simulink model "OFDM_Tx_Rx_InterpDec"  (R2020a)
settings: Solver=FixedStepDiscrete  StartTime=0.0  StopTime=inf  RelTol=1e-3
InitFcn:
  | % Set parameters
  | fs = 200e3;
  | 
  | % Load all required variables
  | load('read_addr_data');
  | load('read_addr_cp');
  | load('read_addr_pream');
  | load('read_addr_rx');
  | load('pilot');
  | load('LTSfreq');
  | load('STSfreq');
  | load('LTSread');
  | load('STSread');
  | load('bpsk');
  | load('qpsk');
  | load('qam16');
values from neighbouring files (symbols this model uses):
  bpsk = [0 0 1 1 1 1 0 0 1 0 1 0 ... (48 elements, 48x1)]    [bpsk.mat]
  qam16 = [12 5 10 3 14 8 1 10 8 7 2 13 ... (48 elements, 48x1)]    [qam16.mat]
  qpsk = [1 2 1 2 2 2 3 1 1 3 1 0 ... (48 elements, 48x1)]    [qpsk.mat]
  STSfreq = [0 0 0 0 0 0 0 0 1 0 0 0 ... (64 elements, 1x64)]    [STSfreq.mat]
undefined symbols (not defined in the file or in its folder): data3, designMultirateFIR, LTSfreq, LTSread, pilot, read_addr_cp, read_addr_data, read_addr_pream, read_addr_rx, STSread
libraries: hdlsllib x58, simulink x42, dspmlti4 x8, dsphdlxfrm x2, dsphdlmathfun x2, dsphdlsigops x1
(part 2 of 5)

== system OFDM_Tx_Rx_InterpDec/OFDMTx/ControlSignalGenerator/pilotValidGen ==
  enb : Inport
  AND : Logic  IconShape=distinctive  AllPortsSameDT=off  OutDataTypeStr=boolean
  Compare To Constant : simulink/Logic and Bit Operations/Compare To Constant  relop=<  const=32  OutDataTypeStr=boolean
  Compare To Constant1 : simulink/Logic and Bit Operations/Compare To Constant  relop=>  const=27  OutDataTypeStr=boolean
  HDL Counter : hdlsllib/Sources/HDL Counter  CountType=Count limited  CountInit=0  CountStep=1  CountMax=79  CountFromType=Initial value  CountFrom=0  CountResetPort=on  CountLoadPort=off  CountEnbPort=on  CountDirPort=off  CountDataType=Unsigned  CountWordLen=7  CountFracLen=0  CountSampTime=1
  NOT : Logic  Operator=NOT  IconShape=distinctive  AllPortsSameDT=off  OutDataTypeStr=boolean
  y : Outport
  wires:
  NOT/1 -> HDL Counter/1
  enb/1 -> HDL Counter/2, NOT/1
  HDL Counter/1 -> Compare To Constant1/1, Compare To Constant/1
  Compare To Constant/1 -> AND/1
  Compare To Constant1/1 -> AND/2
  AND/1 -> y/1

== system OFDM_Tx_Rx_InterpDec/OFDMTx/DataGenerator/LTSfreq ==
  preambVal : Inport
  AND : Logic  IconShape=distinctive  AllPortsSameDT=off  OutDataTypeStr=boolean
  AND1 : Logic  IconShape=distinctive  AllPortsSameDT=off  OutDataTypeStr=boolean
  Compare To Constant : simulink/Logic and Bit Operations/Compare To Constant  relop=>=  const=256  OutDataTypeStr=boolean
  Compare To Constant1 : simulink/Logic and Bit Operations/Compare To Constant  relop=<=  const=319  OutDataTypeStr=boolean
  HDL Counter1 : hdlsllib/Sources/HDL Counter  CountType=Count limited  CountInit=0  CountStep=1  CountMax=319  CountFromType=Initial value  CountFrom=0  CountResetPort=on  CountLoadPort=off  CountEnbPort=on  CountDirPort=off  CountDataType=Unsigned  CountWordLen=9  CountFracLen=0  CountSampTime=1
  HDL Counter4 : hdlsllib/Sources/HDL Counter  CountType=Count limited  CountInit=0  CountStep=1  CountMax=63  CountFromType=Initial value  CountFrom=0  CountResetPort=off  CountLoadPort=off  CountEnbPort=on  CountDirPort=off  CountDataType=Unsigned  CountWordLen=6  CountFracLen=0  CountSampTime=1
  LTSFreq : Lookup_n-D  NumberOfTableDimensions=1  LookupTableObject=''  BreakpointsForDimension1=0:63  BreakpointsForDimension1FirstPoint=10  BreakpointsForDimension2FirstPoint=10  BreakpointsForDimension1Spacing=12  BreakpointsForDimension2Spacing=12  IndexSearchMethod=Evenly spaced points  Table=LTSfreq  TableDataTypeStr=fixdt(1,16,14)  InterpMethod=Flat  DiagnosticForOutOfRangeInput=Error  InternalRulePriority=Speed  OutDataTypeStr=fixdt(1,16,14)  RndMeth=Simplest  InputSameDT=on
  NOT : Logic  Operator=NOT  IconShape=distinctive  AllPortsSameDT=off  OutDataTypeStr=boolean
  ltsFreq : Outport  VectorParamsAs1DForOutWhenUnconnected=off
  ltsVal : Outport  Port=2  VectorParamsAs1DForOutWhenUnconnected=off
  wires:
  HDL Counter4/1 -> LTSFreq/1
  Compare To Constant/1 -> AND/1
  HDL Counter1/1 -> Compare To Constant1/1, Compare To Constant/1
  Compare To Constant1/1 -> AND/2
  NOT/1 -> HDL Counter1/1
  AND/1 -> AND1/1
  preambVal/1 -> NOT/1, AND1/2, HDL Counter1/2
  AND1/1 -> ltsVal/1, HDL Counter4/1
  LTSFreq/1 -> ltsFreq/1

== system OFDM_Tx_Rx_InterpDec/OFDMTx/DataGenerator/PilotGen ==
  dataValidIn : Inport
  pilotValidIn : Inport  Port=2
  Compare To Constant : simulink/Logic and Bit Operations/Compare To Constant  relop=>  const=0  OutDataTypeStr=boolean
  Compare To Constant1 : simulink/Logic and Bit Operations/Compare To Constant  relop===  const=79  OutDataTypeStr=boolean
  Constant : Constant  Value=0  OutDataTypeStr=fixdt(1,2,0)  SampleTime=1/fs
  Data Type Conversion1 : DataTypeConversion  OutDataTypeStr=fixdt(1,16,14)
  HDL Counter : hdlsllib/Sources/HDL Counter  CountType=Count limited  CountInit=0  CountStep=1  CountMax=3  CountFromType=Initial value  CountFrom=0  CountResetPort=off  CountLoadPort=off  CountEnbPort=on  CountDirPort=off  CountDataType=Unsigned  CountWordLen=2  CountFracLen=0  CountSampTime=1
  HDL Counter1 : hdlsllib/Sources/HDL Counter  CountType=Count limited  CountInit=0  CountStep=1  CountMax=79  CountFromType=Initial value  CountFrom=0  CountResetPort=on  CountLoadPort=off  CountEnbPort=on  CountDirPort=off  CountDataType=Unsigned  CountWordLen=8  CountFracLen=0  CountSampTime=1
  HDL Counter2 : hdlsllib/Sources/HDL Counter  CountType=Count limited  CountInit=0  CountStep=1  CountMax=126  CountFromType=Initial value  CountFrom=0  CountResetPort=on  CountLoadPort=off  CountEnbPort=on  CountDirPort=off  CountDataType=Unsigned  CountWordLen=7  CountFracLen=0  CountSampTime=1
  NOT : Logic  Operator=NOT  IconShape=distinctive  AllPortsSameDT=off  OutDataTypeStr=boolean
  PilotValue_LUT : Lookup_n-D  NumberOfTableDimensions=1  LookupTableObject=''  BreakpointsForDimension1=[0:3]  BreakpointsForDimension1FirstPoint=10  BreakpointsForDimension2FirstPoint=10  BreakpointsForDimension1Spacing=12  BreakpointsForDimension2Spacing=12  IndexSearchMethod=Evenly spaced points  Table=[1 1 1 -1]  TableDataTypeStr=fixdt(1,2,0)  InterpMethod=Flat  DiagnosticForOutOfRangeInput=Error  InternalRulePriority=Speed  OutDataTypeStr=fixdt(1,2,0)  RndMeth=Simplest  InputSameDT=on
  Polarity_LUT : Lookup_n-D  NumberOfTableDimensions=1  LookupTableObject=''  BreakpointsForDimension1=[0:126]  BreakpointsForDimension1FirstPoint=10  BreakpointsForDimension2FirstPoint=10  BreakpointsForDimension1Spacing=12  BreakpointsForDimension2Spacing=12  IndexSearchMethod=Evenly spaced points  Table=pilot  TableDataTypeStr=fixdt(1,2,0)  InterpMethod=Flat  DiagnosticForOutOfRangeInput=Error  InternalRulePriority=Speed  OutDataTypeStr=fixdt(1,2,0)  RndMeth=Simplest  InputSameDT=on
  Switch : Switch  Criteria=u2 ~= 0
  Switch1 : Switch  Criteria=u2 ~= 0
  ToComplex1 : Subsystem
  Unary Minus : UnaryMinus
  pilotOut : Outport  VectorParamsAs1DForOutWhenUnconnected=off
  wires:
  HDL Counter/1 -> PilotValue_LUT/1
  Data Type Conversion1/1 -> ToComplex1/1(In1)
  dataValidIn/1 -> HDL Counter1/2, NOT/1
  HDL Counter1/1 -> Compare To Constant1/1
  NOT/1 -> HDL Counter2/1, HDL Counter1/1
  Compare To Constant1/1 -> HDL Counter2/2
  HDL Counter2/1 -> Polarity_LUT/1
  ToComplex1/1(PilotOut) -> pilotOut/1
  pilotValidIn/1 -> HDL Counter/1, Switch1/2
  Polarity_LUT/1 -> Compare To Constant/1
  Compare To Constant/1 -> Switch/2
  Unary Minus/1 -> Switch/3
  Switch/1 -> Data Type Conversion1/1
  PilotValue_LUT/1 -> Switch1/1
  Switch1/1 -> Unary Minus/1, Switch/1
  Constant/1 -> Switch1/3

== system OFDM_Tx_Rx_InterpDec/OFDMTx/DataGenerator/STSFreq ==
  preamVal : Inport
  AND : Logic  IconShape=distinctive  AllPortsSameDT=off  OutDataTypeStr=boolean
  AND1 : Logic  IconShape=distinctive  AllPortsSameDT=off  OutDataTypeStr=boolean
  Compare To Constant : simulink/Logic and Bit Operations/Compare To Constant  relop=>=  const=96  OutDataTypeStr=boolean
  Compare To Constant1 : simulink/Logic and Bit Operations/Compare To Constant  relop=<=  const=159  OutDataTypeStr=boolean
  HDL Counter : hdlsllib/Sources/HDL Counter  CountType=Count limited  CountInit=0  CountStep=1  CountMax=63  CountFromType=Initial value  CountFrom=0  CountResetPort=off  CountLoadPort=off  CountEnbPort=on  CountDirPort=off  CountDataType=Unsigned  CountWordLen=6  CountFracLen=0  CountSampTime=1
  HDL Counter1 : hdlsllib/Sources/HDL Counter  CountType=Count limited  CountInit=0  CountStep=1  CountMax=319  CountFromType=Initial value  CountFrom=0  CountResetPort=on  CountLoadPort=off  CountEnbPort=on  CountDirPort=off  CountDataType=Unsigned  CountWordLen=9  CountFracLen=0  CountSampTime=1
  NOT : Logic  Operator=NOT  IconShape=distinctive  AllPortsSameDT=off  OutDataTypeStr=boolean
  STSFreq : Lookup_n-D  NumberOfTableDimensions=1  LookupTableObject=''  BreakpointsForDimension1=[0:63]  BreakpointsForDimension1FirstPoint=10  BreakpointsForDimension2FirstPoint=10  BreakpointsForDimension1Spacing=12  BreakpointsForDimension2Spacing=12  IndexSearchMethod=Evenly spaced points  Table=STSfreq  TableDataTypeStr=fixdt(1,16,14)  InterpMethod=Flat  DiagnosticForOutOfRangeInput=Error  InternalRulePriority=Speed  OutDataTypeStr=fixdt(1,16,14)  RndMeth=Simplest  InputSameDT=on
  stsFreq : Outport  VectorParamsAs1DForOutWhenUnconnected=off
  stsVal : Outport  Port=2  VectorParamsAs1DForOutWhenUnconnected=off
  wires:
  HDL Counter/1 -> STSFreq/1
  AND/1 -> AND1/1
  HDL Counter1/1 -> Compare To Constant1/1, Compare To Constant/1
  NOT/1 -> HDL Counter1/1
  Compare To Constant/1 -> AND/1
  Compare To Constant1/1 -> AND/2
  preamVal/1 -> NOT/1, AND1/2, HDL Counter1/2
  AND1/1 -> stsVal/1, HDL Counter/1
  STSFreq/1 -> stsFreq/1

== system OFDM_Tx_Rx_InterpDec/OFDMTx/DataGenerator/SymbolsGen ==
  modScheme : Inport
  valid : Inport  Port=2
  BPSKmap : Subsystem
  DataGenerator : Subsystem
  DataGenerator1 : Subsystem
  DataGenerator2 : Subsystem  Commented=on
  DataGenerator3 : Subsystem
  Multiport Switch : MultiPortSwitch  DataPortOrder=Zero-based contiguous  zeroidx=on
  QPSKMap : Subsystem
  QPSKMap1 : Subsystem
  symbsOut : Outport  VectorParamsAs1DForOutWhenUnconnected=off
  wires:
  BPSKmap/1(BPSKOut) -> Multiport Switch/2
  modScheme/1 -> Multiport Switch/1
  Multiport Switch/1 -> symbsOut/1
  QPSKMap/1(QPSKOut) -> Multiport Switch/3
  QPSKMap1/1(16QAM) -> Multiport Switch/4
  DataGenerator3/1(bits) -> QPSKMap1/1(ints)
  DataGenerator3/2(validOut) -> QPSKMap1/2(validIn)
  DataGenerator1/1(bits) -> QPSKMap/1(ints)
  DataGenerator1/2(validOut) -> QPSKMap/2(validIn)
  DataGenerator/1(bits) -> BPSKmap/1(bits)
  DataGenerator/2(validOut) -> BPSKmap/2(validIn)
  valid/1 -> DataGenerator3/1(ready), DataGenerator1/1(ready), DataGenerator/1(ready)

== system OFDM_Tx_Rx_InterpDec/OFDMTx/IFFT/IFFTValid ==
  preambleValid : Inport
  dataValid : Inport  Port=2
  Switch : Switch  Criteria=u2 ~= 0
  dataIFFTValid : Subsystem
  preambIFFTValid : Subsystem
  ifftValid : Outport  VectorParamsAs1DForOutWhenUnconnected=off
  wires:
  preambleValid/1 -> Switch/2, preambIFFTValid/1(preambValid)
  preambIFFTValid/1(preambIFFTValidOut) -> Switch/1
  dataValid/1 -> dataIFFTValid/1(dataValidIn)
  dataIFFTValid/1(dataIFFTValidOut) -> Switch/3
  Switch/1 -> ifftValid/1

== system OFDM_Tx_Rx_InterpDec/OFDMTx/SCMapper/DataMapper ==
  dataIn : Inport
  dataValid : Inport  Port=2
  Delay1 : Delay  DelayLength=80  InitialCondition=0  UseCircularBuffer=on
  Delay2 : Delay  DelayLength=80
  Delay3 : Delay  DelayLength=1  InitialCondition=0  UseCircularBuffer=on
  Delay4 : Delay  DelayLength=80
  Dual Port RAM2 : hdlsllib/HDL RAMs/Dual Port RAM  ram_size=8
      settings: SourceProductBaseCode=SL
  HDL Counter : hdlsllib/Sources/HDL Counter  CountType=Count limited  CountInit=0  CountStep=1  CountMax=159  CountFromType=Initial value  CountFrom=0  CountResetPort=off  CountLoadPort=off  CountEnbPort=on  CountDirPort=off  CountDataType=Unsigned  CountWordLen=8  CountFracLen=0  CountSampTime=1
  HDL Counter1 : hdlsllib/Sources/HDL Counter  CountType=Count limited  CountInit=0  CountStep=1  CountMax=159  CountFromType=Initial value  CountFrom=0  CountResetPort=off  CountLoadPort=off  CountEnbPort=on  CountDirPort=off  CountDataType=Unsigned  CountWordLen=8  CountFracLen=0  CountSampTime=1
  READ_CTRL2 : Subsystem
  Terminator3 : Terminator
  readaddress : Lookup_n-D  NumberOfTableDimensions=1  LookupTableObject=''  BreakpointsForDimension1=[0:159]  BreakpointsForDimension1FirstPoint=10  BreakpointsForDimension2FirstPoint=10  BreakpointsForDimension1Spacing=12  BreakpointsForDimension2Spacing=12  IndexSearchMethod=Evenly spaced points  Table=read_addr_data  TableDataTypeStr=fixdt(0,8,0)  InterpMethod=Flat  DiagnosticForOutOfRangeInput=Error  InternalRulePriority=Speed  OutDataTypeStr=fixdt(0,8,0)  RndMeth=Simplest  InputSameDT=on
  dataOut : Outport  VectorParamsAs1DForOutWhenUnconnected=off
  dataValidOut : Outport  Port=2  VectorParamsAs1DForOutWhenUnconnected=off
  wires:
  READ_CTRL2/1(Out1) -> Dual Port RAM2/4
  Delay3/1 -> Delay2/1
  dataValid/1 -> HDL Counter1/1, Delay1/1, Dual Port RAM2/3
  Dual Port RAM2/2 -> Delay4/1
  Delay1/1 -> READ_CTRL2/2(In2), Delay3/1, HDL Counter/1
  HDL Counter1/1 -> Dual Port RAM2/2
  dataIn/1 -> Dual Port RAM2/1
  HDL Counter/1 -> readaddress/1
  readaddress/1 -> READ_CTRL2/1(In1)
  Dual Port RAM2/1 -> Terminator3/1
  Delay2/1 -> dataValidOut/1
  Delay4/1 -> dataOut/1

== system OFDM_Tx_Rx_InterpDec/OFDMTx/SCMapper/PremableMapper ==
  data : Inport
  preambVal : Inport  Port=2
  Delay : Delay  DelayLength=160  InitialCondition=0  UseCircularBuffer=on
  Delay12 : Delay  DelayLength=1  InitialCondition=0  UseCircularBuffer=on
  Dual Port RAM : hdlsllib/HDL RAMs/Dual Port RAM  ram_size=9
      settings: SourceProductBaseCode=SL
  HDL Counter2 : hdlsllib/Sources/HDL Counter  CountType=Count limited  CountInit=0  CountStep=1  CountMax=319  CountFromType=Initial value  CountFrom=0  CountResetPort=off  CountLoadPort=off  CountEnbPort=on  CountDirPort=off  CountDataType=Unsigned  CountWordLen=9  CountFracLen=0  CountSampTime=1
  HDL Counter3 : hdlsllib/Sources/HDL Counter  CountType=Count limited  CountInit=0  CountStep=1  CountMax=319  CountFromType=Initial value  CountFrom=0  CountResetPort=off  CountLoadPort=off  CountEnbPort=on  CountDirPort=off  CountDataType=Unsigned  CountWordLen=9  CountFracLen=0  CountSampTime=1
  READ_CTRL : Subsystem
  Terminator1 : Terminator
  readaddr : Lookup_n-D  NumberOfTableDimensions=1  LookupTableObject=''  BreakpointsForDimension1=0:319  BreakpointsForDimension1FirstPoint=10  BreakpointsForDimension2FirstPoint=10  BreakpointsForDimension1Spacing=12  BreakpointsForDimension2Spacing=12  IndexSearchMethod=Evenly spaced points  Table=read_addr_pream  TableDataTypeStr=fixdt(0,9,0)  InterpMethod=Flat  DiagnosticForOutOfRangeInput=Error  InternalRulePriority=Speed  OutDataTypeStr=fixdt(0,9,0)  RndMeth=Simplest  InputSameDT=on
  preambleShiftOut : Outport  VectorParamsAs1DForOutWhenUnconnected=off
  preambValOut : Outport  Port=2  VectorParamsAs1DForOutWhenUnconnected=off
  wires:
  readaddr/1 -> READ_CTRL/1(In1)
  preambVal/1 -> Delay/1, Dual Port RAM/3, HDL Counter3/1
  READ_CTRL/1(Out1) -> Dual Port RAM/4
  HDL Counter3/1 -> Dual Port RAM/2
  Delay/1 -> READ_CTRL/2(In2), Delay12/1, HDL Counter2/1
  Dual Port RAM/1 -> Terminator1/1
  Delay12/1 -> preambValOut/1
  HDL Counter2/1 -> readaddr/1
  data/1 -> Dual Port RAM/1
  Dual Port RAM/2 -> preambleShiftOut/1

== system OFDM_Tx_Rx_InterpDec/OFDMRx/ChannelEstEq/ChannelEstimate/ChanEst ==
  note: Store conjugate as this is used in the
      | equaliser.
  note: Read out frequency domain LTS
      | when preamble valid is HIGH and
      | use this to obtain channel estimate.
  note: 1st half
  note: 2nd half
  ChanEstIn : Inport
  PreambValidIn : Inport  Port=2
  Delay : Delay  DelayLength=64
  Delay{1..7} (7 alike) : Delay  DelayLength=1
  Gain : Gain  Gain=0.5  OutDataTypeStr=fixdt(1,17,14)
  HDL Counter : hdlsllib/Sources/HDL Counter  CountType=Count limited  CountInit=0  CountStep=1  CountMax=63  CountFromType=Initial value  CountFrom=0  CountResetPort=off  CountLoadPort=off  CountEnbPort=on  CountDirPort=off  CountDataType=Unsigned  CountWordLen=6  CountFracLen=0  CountSampTime=1
  InvLLTF : Lookup_n-D  NumberOfTableDimensions=1  BreakpointsForDimension1=0:63  IndexSearchMethod=Evenly spaced points  Table=fftshift(LTSfreq)  TableDataTypeStr=fixdt(1,16,0)  InterpMethod=Flat  ExtrapMethod=Clip  UseLastTableValue=on  InternalRulePriority=Speed  OutDataTypeStr=fixdt(1,16,0)  RndMeth=Simplest  InputSameDT=on
  Math Function : Math  Operator=conj  SignedPower=on  SaturateOnIntegerOverflow=on
  Product : Product  OutDataTypeStr=fixdt(1,16,14)
  Subtract : Sum
  ChEstOut : Outport  VectorParamsAs1DForOutWhenUnconnected=off
  wires:
  Delay7/1 -> Math Function/1
  Delay6/1 -> Subtract/2, Delay/1
  Delay5/1 -> Product/2
  InvLLTF/1 -> Delay5/1
  Delay4/1 -> Product/1
  HDL Counter/1 -> InvLLTF/1
  Gain/1 -> Delay7/1
  Product/1 -> Delay6/1
  Delay/1 -> Subtract/1
  Math Function/1 -> Delay3/1
  ChanEstIn/1 -> Delay1/1
  PreambValidIn/1 -> Delay2/1
  Delay1/1 -> Delay4/1
  Delay2/1 -> HDL Counter/1
  Delay3/1 -> ChEstOut/1
  Subtract/1 -> Gain/1

== system OFDM_Tx_Rx_InterpDec/OFDMRx/ChannelEstEq/ChannelEstimate/WriteEnbAddrGen ==
  In1 : Inport
  AND : Logic  IconShape=distinctive  AllPortsSameDT=off  OutDataTypeStr=boolean
  Compare To Constant : simulink/Logic and Bit Operations/Compare To Constant  relop=>=  const=64  OutDataTypeStr=boolean
  Compare To Constant1 : simulink/Logic and Bit Operations/Compare To Constant  relop=<=  const=127  OutDataTypeStr=boolean
  HDL Counter1 : hdlsllib/Sources/HDL Counter  CountType=Count limited  CountInit=0  CountStep=1  CountMax=63  CountFromType=Initial value  CountFrom=0  CountResetPort=off  CountLoadPort=off  CountEnbPort=on  CountDirPort=off  CountDataType=Unsigned  CountWordLen=6  CountFracLen=0  CountSampTime=1
  HDL Counter2 : hdlsllib/Sources/HDL Counter  CountType=Count limited  CountInit=0  CountStep=1  CountMax=127  CountFromType=Initial value  CountFrom=0  CountResetPort=off  CountLoadPort=off  CountEnbPort=on  CountDirPort=off  CountDataType=Unsigned  CountWordLen=7  CountFracLen=0  CountSampTime=1
  Out1 : Outport  VectorParamsAs1DForOutWhenUnconnected=off
  Out2 : Outport  Port=2  VectorParamsAs1DForOutWhenUnconnected=off
  wires:
  In1/1 -> HDL Counter2/1
  HDL Counter2/1 -> Compare To Constant/1, Compare To Constant1/1
  AND/1 -> Out2/1, HDL Counter1/1
  HDL Counter1/1 -> Out1/1
  Compare To Constant/1 -> AND/1
  Compare To Constant1/1 -> AND/2

== system OFDM_Tx_Rx_InterpDec/OFDMRx/ChannelEstEq/Equalise/Abs2 ==
  ChEstIn : Inport
  Add : Sum  OutDataTypeStr=fixdt(0,16,14)
  Complex to Real-Imag : ComplexToRealImag
  Delay{,1..4} (5 alike) : Delay  DelayLength=1
  Product : Product
  Product1 : Product
  Out1 : Outport  VectorParamsAs1DForOutWhenUnconnected=off
  wires:
  Delay3/1 -> Add/2
  Delay2/1 -> Add/1
  Delay1/1 -> Product1/1, Product1/2
  Delay/1 -> Product/2, Product/1
  Complex to Real-Imag/2 -> Delay1/1
  Product1/1 -> Delay3/1
  Product/1 -> Delay2/1
  ChEstIn/1 -> Complex to Real-Imag/1
  Complex to Real-Imag/1 -> Delay/1
  Add/1 -> Delay4/1
  Delay4/1 -> Out1/1

== system OFDM_Tx_Rx_InterpDec/OFDMRx/ChannelEstEq/Equalise/Complex Mult ==
  In1 : Inport
  In2 : Inport  Port=2
  Delay4 : Delay  DelayLength=1
  Delay5 : Delay  DelayLength=1
  Delay7 : Delay
  Product1 : Product  OutDataTypeStr=fixdt(1,18,15)
  Out1 : Outport
  wires:
  Product1/1 -> Delay7/1
  Delay4/1 -> Product1/1
  In1/1 -> Delay4/1
  Delay5/1 -> Product1/2
  Delay7/1 -> Out1/1
  In2/1 -> Delay5/1

== system OFDM_Tx_Rx_InterpDec/OFDMRx/ChannelEstEq/Equalise/Divide ==
  In1 : Inport
  In2 : Inport  Port=2
  Delay1 : Delay  DelayLength=1
  Delay2 : Delay  DelayLength=1
  Delay8 : Delay  DelayLength=1
  Product2 : Product  OutDataTypeStr=fixdt(1,18,15)
  Reciprocal : Product  Inputs=/  OutDataTypeStr=fixdt(0,25,15)  RndMeth=Zero  SaturateOnIntegerOverflow=on
  Out1 : Outport
  wires:
  Reciprocal/1 -> Delay1/1
  In2/1 -> Reciprocal/1
  In1/1 -> Delay8/1
  Delay8/1 -> Product2/1
  Delay1/1 -> Product2/2
  Product2/1 -> Delay2/1
  Delay2/1 -> Out1/1

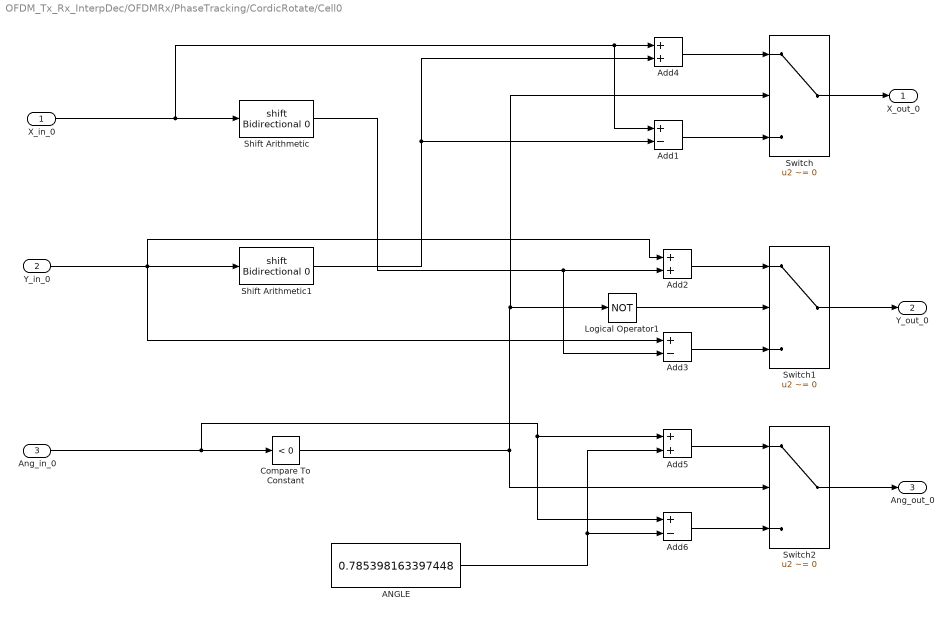
== system OFDM_Tx_Rx_InterpDec/OFDMRx/PhaseTracking/CordicRotate/Cell0 ==
  X_in_0 : Inport
  Y_in_0 : Inport  Port=2
  Ang_in_0 : Inport  Port=3
  ANGLE : Constant  Value=0.785398163397448  VectorParams1D=off  OutDataTypeStr=fixdt(1,23,20)  SampleTime=1/fs
  Add1 : Sum  Inputs=+-  OutDataTypeStr=fixdt(1,21,15)
  Add2 : Sum  OutDataTypeStr=fixdt(1,21,15)
  Add3 : Sum  Inputs=+-  OutDataTypeStr=fixdt(1,21,15)
  Add4 : Sum  OutDataTypeStr=fixdt(1,21,15)
  Add5 : Sum  OutDataTypeStr=fixdt(1,23,20)
  Add6 : Sum  Inputs=+-  OutDataTypeStr=fixdt(1,23,20)
  Compare To Constant : simulink/Logic and Bit Operations/Compare To Constant  relop=<  const=0  OutDataTypeStr=boolean
  Logical Operator1 : Logic  Operator=NOT  IconShape=distinctive  AllPortsSameDT=off  OutDataTypeStr=boolean
  Shift Arithmetic : ArithShift
  Shift Arithmetic1 : ArithShift
  Switch : Switch  Criteria=u2 ~= 0
  Switch1 : Switch  Criteria=u2 ~= 0
  Switch2 : Switch  Criteria=u2 ~= 0
  X_out_0 : Outport  VectorParamsAs1DForOutWhenUnconnected=off
  Y_out_0 : Outport  Port=2  VectorParamsAs1DForOutWhenUnconnected=off
  Ang_out_0 : Outport  Port=3  VectorParamsAs1DForOutWhenUnconnected=off
  wires:
  ANGLE/1 -> Add5/2, Add6/2
  Logical Operator1/1 -> Switch1/2
  Shift Arithmetic/1 -> Add2/2, Add3/2
  Shift Arithmetic1/1 -> Add4/2, Add1/2
  Compare To Constant/1 -> Switch2/2, Switch/2, Logical Operator1/1
  Ang_in_0/1 -> Compare To Constant/1, Add5/1, Add6/1
  Y_in_0/1 -> Add2/1, Add3/1, Shift Arithmetic1/1
  X_in_0/1 -> Add4/1, Add1/1, Shift Arithmetic/1
  Switch2/1 -> Ang_out_0/1
  Add5/1 -> Switch2/1
  Add6/1 -> Switch2/3
  Switch1/1 -> Y_out_0/1
  Switch/1 -> X_out_0/1
  Add2/1 -> Switch1/1
  Add3/1 -> Switch1/3
  Add1/1 -> Switch/3
  Add4/1 -> Switch/1

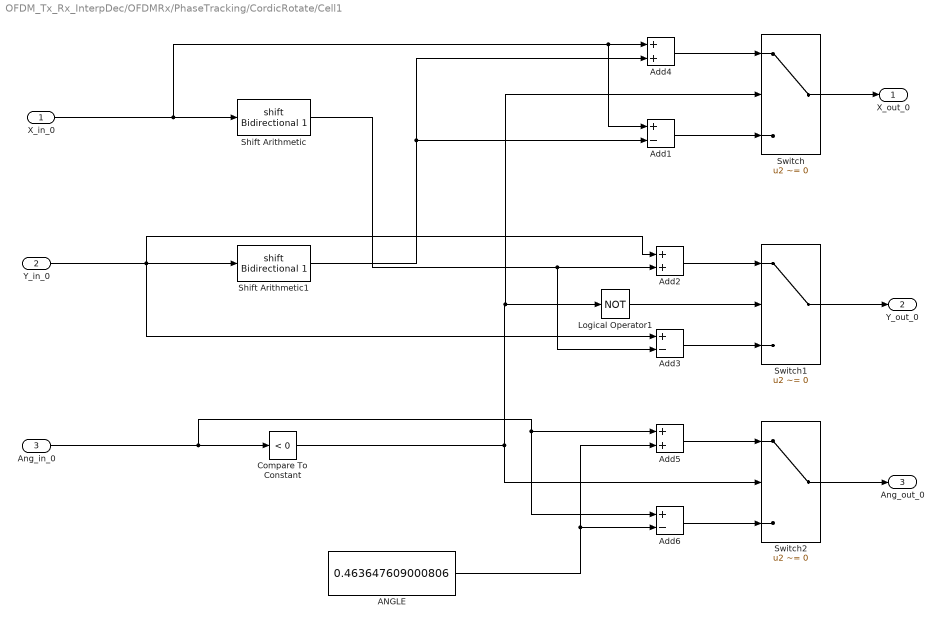
== system OFDM_Tx_Rx_InterpDec/OFDMRx/PhaseTracking/CordicRotate/Cell1 ==
  X_in_0 : Inport
  Y_in_0 : Inport  Port=2
  Ang_in_0 : Inport  Port=3
  ANGLE : Constant  Value=0.463647609000806  VectorParams1D=off  OutDataTypeStr=fixdt(1,23,20)  SampleTime=1/fs
  Add1 : Sum  Inputs=+-  OutDataTypeStr=fixdt(1,21,15)
  Add2 : Sum  OutDataTypeStr=fixdt(1,21,15)
  Add3 : Sum  Inputs=+-  OutDataTypeStr=fixdt(1,21,15)
  Add4 : Sum  OutDataTypeStr=fixdt(1,21,15)
  Add5 : Sum  OutDataTypeStr=fixdt(1,23,20)
  Add6 : Sum  Inputs=+-  OutDataTypeStr=fixdt(1,23,20)
  Compare To Constant : simulink/Logic and Bit Operations/Compare To Constant  relop=<  const=0  OutDataTypeStr=boolean
  Logical Operator1 : Logic  Operator=NOT  IconShape=distinctive  AllPortsSameDT=off  OutDataTypeStr=boolean
  Shift Arithmetic : ArithShift  BitShiftNumber=1
  Shift Arithmetic1 : ArithShift  BitShiftNumber=1
  Switch : Switch  Criteria=u2 ~= 0
  Switch1 : Switch  Criteria=u2 ~= 0
  Switch2 : Switch  Criteria=u2 ~= 0
  X_out_0 : Outport  VectorParamsAs1DForOutWhenUnconnected=off
  Y_out_0 : Outport  Port=2  VectorParamsAs1DForOutWhenUnconnected=off
  Ang_out_0 : Outport  Port=3  VectorParamsAs1DForOutWhenUnconnected=off
  wires:
  Add4/1 -> Switch/1
  Add1/1 -> Switch/3
  Add3/1 -> Switch1/3
  Add2/1 -> Switch1/1
  Switch/1 -> X_out_0/1
  Switch1/1 -> Y_out_0/1
  Add6/1 -> Switch2/3
  Add5/1 -> Switch2/1
  Switch2/1 -> Ang_out_0/1
  X_in_0/1 -> Shift Arithmetic/1, Add1/1, Add4/1
  Y_in_0/1 -> Shift Arithmetic1/1, Add3/1, Add2/1
  Ang_in_0/1 -> Add6/1, Add5/1, Compare To Constant/1
  Compare To Constant/1 -> Logical Operator1/1, Switch/2, Switch2/2
  Shift Arithmetic1/1 -> Add1/2, Add4/2
  Shift Arithmetic/1 -> Add3/2, Add2/2
  Logical Operator1/1 -> Switch1/2
  ANGLE/1 -> Add6/2, Add5/2

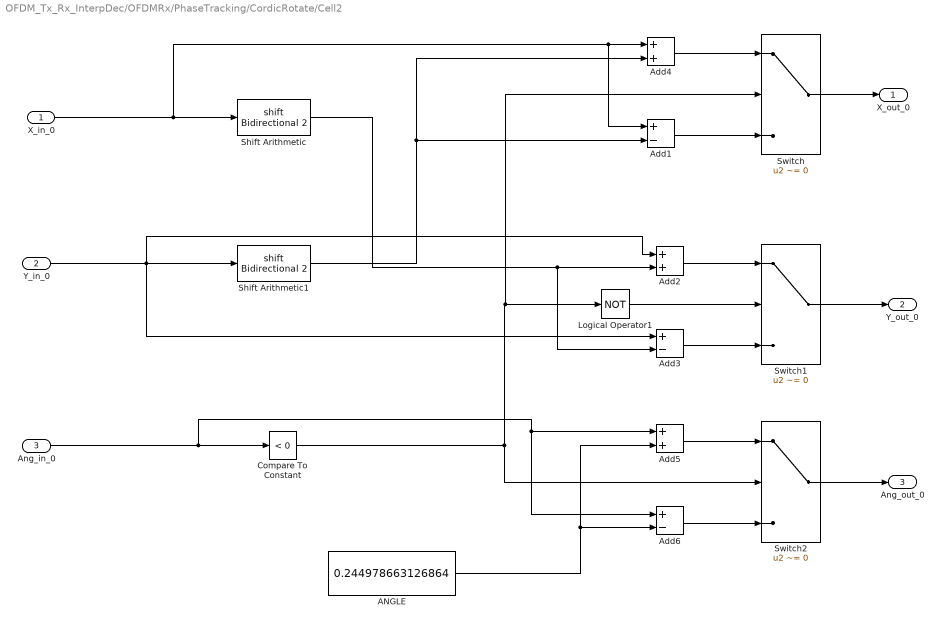
== system OFDM_Tx_Rx_InterpDec/OFDMRx/PhaseTracking/CordicRotate/Cell2 ==
  X_in_0 : Inport
  Y_in_0 : Inport  Port=2
  Ang_in_0 : Inport  Port=3
  ANGLE : Constant  Value=0.244978663126864  VectorParams1D=off  OutDataTypeStr=fixdt(1,23,20)  SampleTime=1/fs
  Add1 : Sum  Inputs=+-  OutDataTypeStr=fixdt(1,21,15)
  Add2 : Sum  OutDataTypeStr=fixdt(1,21,15)
  Add3 : Sum  Inputs=+-  OutDataTypeStr=fixdt(1,21,15)
  Add4 : Sum  OutDataTypeStr=fixdt(1,21,15)
  Add5 : Sum  OutDataTypeStr=fixdt(1,23,20)
  Add6 : Sum  Inputs=+-  OutDataTypeStr=fixdt(1,23,20)
  Compare To Constant : simulink/Logic and Bit Operations/Compare To Constant  relop=<  const=0  OutDataTypeStr=boolean
  Logical Operator1 : Logic  Operator=NOT  IconShape=distinctive  AllPortsSameDT=off  OutDataTypeStr=boolean
  Shift Arithmetic : ArithShift  BitShiftNumber=2
  Shift Arithmetic1 : ArithShift  BitShiftNumber=2
  Switch : Switch  Criteria=u2 ~= 0
  Switch1 : Switch  Criteria=u2 ~= 0
  Switch2 : Switch  Criteria=u2 ~= 0
  X_out_0 : Outport  VectorParamsAs1DForOutWhenUnconnected=off
  Y_out_0 : Outport  Port=2  VectorParamsAs1DForOutWhenUnconnected=off
  Ang_out_0 : Outport  Port=3  VectorParamsAs1DForOutWhenUnconnected=off
  wires:
  ANGLE/1 -> Add5/2, Add6/2
  Logical Operator1/1 -> Switch1/2
  Shift Arithmetic/1 -> Add2/2, Add3/2
  Shift Arithmetic1/1 -> Add4/2, Add1/2
  Compare To Constant/1 -> Switch2/2, Switch/2, Logical Operator1/1
  Ang_in_0/1 -> Compare To Constant/1, Add5/1, Add6/1
  Y_in_0/1 -> Add2/1, Add3/1, Shift Arithmetic1/1
  X_in_0/1 -> Add4/1, Add1/1, Shift Arithmetic/1
  Switch2/1 -> Ang_out_0/1
  Add5/1 -> Switch2/1
  Add6/1 -> Switch2/3
  Switch1/1 -> Y_out_0/1
  Switch/1 -> X_out_0/1
  Add2/1 -> Switch1/1
  Add3/1 -> Switch1/3
  Add1/1 -> Switch/3
  Add4/1 -> Switch/1

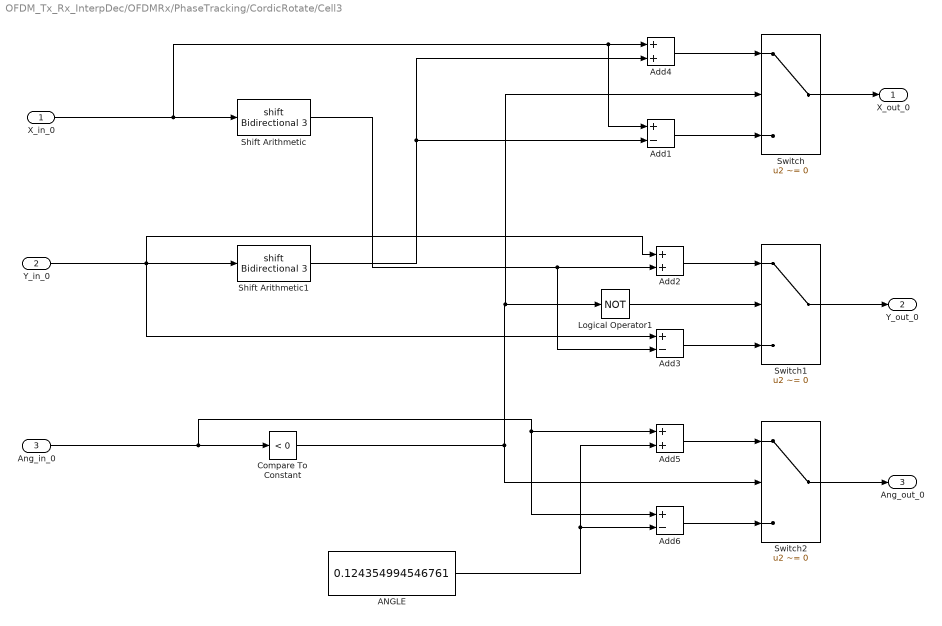
== system OFDM_Tx_Rx_InterpDec/OFDMRx/PhaseTracking/CordicRotate/Cell3 ==
  X_in_0 : Inport
  Y_in_0 : Inport  Port=2
  Ang_in_0 : Inport  Port=3
  ANGLE : Constant  Value=0.124354994546761  VectorParams1D=off  OutDataTypeStr=fixdt(1,23,20)  SampleTime=1/fs
  Add1 : Sum  Inputs=+-  OutDataTypeStr=fixdt(1,21,15)
  Add2 : Sum  OutDataTypeStr=fixdt(1,21,15)
  Add3 : Sum  Inputs=+-  OutDataTypeStr=fixdt(1,21,15)
  Add4 : Sum  OutDataTypeStr=fixdt(1,21,15)
  Add5 : Sum  OutDataTypeStr=fixdt(1,23,20)
  Add6 : Sum  Inputs=+-  OutDataTypeStr=fixdt(1,23,20)
  Compare To Constant : simulink/Logic and Bit Operations/Compare To Constant  relop=<  const=0  OutDataTypeStr=boolean
  Logical Operator1 : Logic  Operator=NOT  IconShape=distinctive  AllPortsSameDT=off  OutDataTypeStr=boolean
  Shift Arithmetic : ArithShift  BitShiftNumber=3
  Shift Arithmetic1 : ArithShift  BitShiftNumber=3
  Switch : Switch  Criteria=u2 ~= 0
  Switch1 : Switch  Criteria=u2 ~= 0
  Switch2 : Switch  Criteria=u2 ~= 0
  X_out_0 : Outport  VectorParamsAs1DForOutWhenUnconnected=off
  Y_out_0 : Outport  Port=2  VectorParamsAs1DForOutWhenUnconnected=off
  Ang_out_0 : Outport  Port=3  VectorParamsAs1DForOutWhenUnconnected=off
  wires:
  Add4/1 -> Switch/1
  Add1/1 -> Switch/3
  Add3/1 -> Switch1/3
  Add2/1 -> Switch1/1
  Switch/1 -> X_out_0/1
  Switch1/1 -> Y_out_0/1
  Add6/1 -> Switch2/3
  Add5/1 -> Switch2/1
  Switch2/1 -> Ang_out_0/1
  X_in_0/1 -> Shift Arithmetic/1, Add1/1, Add4/1
  Y_in_0/1 -> Shift Arithmetic1/1, Add3/1, Add2/1
  Ang_in_0/1 -> Add6/1, Add5/1, Compare To Constant/1
  Compare To Constant/1 -> Logical Operator1/1, Switch/2, Switch2/2
  Shift Arithmetic1/1 -> Add1/2, Add4/2
  Shift Arithmetic/1 -> Add3/2, Add2/2
  Logical Operator1/1 -> Switch1/2
  ANGLE/1 -> Add6/2, Add5/2

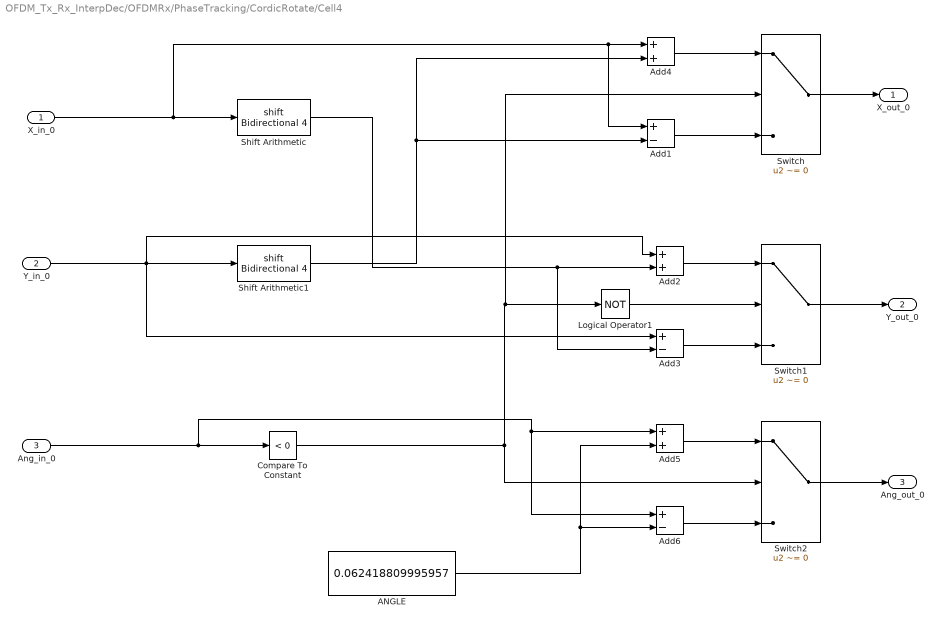
== system OFDM_Tx_Rx_InterpDec/OFDMRx/PhaseTracking/CordicRotate/Cell4 ==
  X_in_0 : Inport
  Y_in_0 : Inport  Port=2
  Ang_in_0 : Inport  Port=3
  ANGLE : Constant  Value=0.062418809995957  VectorParams1D=off  OutDataTypeStr=fixdt(1,23,20)  SampleTime=1/fs
  Add1 : Sum  Inputs=+-  OutDataTypeStr=fixdt(1,21,15)
  Add2 : Sum  OutDataTypeStr=fixdt(1,21,15)
  Add3 : Sum  Inputs=+-  OutDataTypeStr=fixdt(1,21,15)
  Add4 : Sum  OutDataTypeStr=fixdt(1,21,15)
  Add5 : Sum  OutDataTypeStr=fixdt(1,23,20)
  Add6 : Sum  Inputs=+-  OutDataTypeStr=fixdt(1,23,20)
  Compare To Constant : simulink/Logic and Bit Operations/Compare To Constant  relop=<  const=0  OutDataTypeStr=boolean
  Logical Operator1 : Logic  Operator=NOT  IconShape=distinctive  AllPortsSameDT=off  OutDataTypeStr=boolean
  Shift Arithmetic : ArithShift  BitShiftNumber=4
  Shift Arithmetic1 : ArithShift  BitShiftNumber=4
  Switch : Switch  Criteria=u2 ~= 0
  Switch1 : Switch  Criteria=u2 ~= 0
  Switch2 : Switch  Criteria=u2 ~= 0
  X_out_0 : Outport  VectorParamsAs1DForOutWhenUnconnected=off
  Y_out_0 : Outport  Port=2  VectorParamsAs1DForOutWhenUnconnected=off
  Ang_out_0 : Outport  Port=3  VectorParamsAs1DForOutWhenUnconnected=off
  wires:
  ANGLE/1 -> Add5/2, Add6/2
  Logical Operator1/1 -> Switch1/2
  Shift Arithmetic/1 -> Add2/2, Add3/2
  Shift Arithmetic1/1 -> Add4/2, Add1/2
  Compare To Constant/1 -> Switch2/2, Switch/2, Logical Operator1/1
  Ang_in_0/1 -> Compare To Constant/1, Add5/1, Add6/1
  Y_in_0/1 -> Add2/1, Add3/1, Shift Arithmetic1/1
  X_in_0/1 -> Add4/1, Add1/1, Shift Arithmetic/1
  Switch2/1 -> Ang_out_0/1
  Add5/1 -> Switch2/1
  Add6/1 -> Switch2/3
  Switch1/1 -> Y_out_0/1
  Switch/1 -> X_out_0/1
  Add2/1 -> Switch1/1
  Add3/1 -> Switch1/3
  Add1/1 -> Switch/3
  Add4/1 -> Switch/1

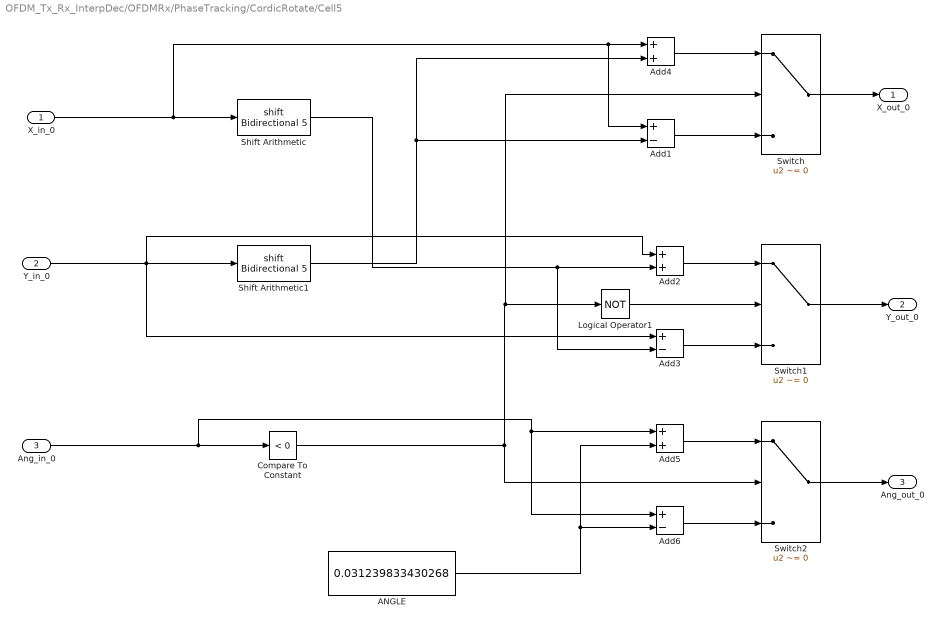
== system OFDM_Tx_Rx_InterpDec/OFDMRx/PhaseTracking/CordicRotate/Cell5 ==
  X_in_0 : Inport
  Y_in_0 : Inport  Port=2
  Ang_in_0 : Inport  Port=3
  ANGLE : Constant  Value=0.031239833430268  VectorParams1D=off  OutDataTypeStr=fixdt(1,23,20)  SampleTime=1/fs
  Add1 : Sum  Inputs=+-  OutDataTypeStr=fixdt(1,21,15)
  Add2 : Sum  OutDataTypeStr=fixdt(1,21,15)
  Add3 : Sum  Inputs=+-  OutDataTypeStr=fixdt(1,21,15)
  Add4 : Sum  OutDataTypeStr=fixdt(1,21,15)
  Add5 : Sum  OutDataTypeStr=fixdt(1,23,20)
  Add6 : Sum  Inputs=+-  OutDataTypeStr=fixdt(1,23,20)
  Compare To Constant : simulink/Logic and Bit Operations/Compare To Constant  relop=<  const=0  OutDataTypeStr=boolean
  Logical Operator1 : Logic  Operator=NOT  IconShape=distinctive  AllPortsSameDT=off  OutDataTypeStr=boolean
  Shift Arithmetic : ArithShift  BitShiftNumber=5
  Shift Arithmetic1 : ArithShift  BitShiftNumber=5
  Switch : Switch  Criteria=u2 ~= 0
  Switch1 : Switch  Criteria=u2 ~= 0
  Switch2 : Switch  Criteria=u2 ~= 0
  X_out_0 : Outport  VectorParamsAs1DForOutWhenUnconnected=off
  Y_out_0 : Outport  Port=2  VectorParamsAs1DForOutWhenUnconnected=off
  Ang_out_0 : Outport  Port=3  VectorParamsAs1DForOutWhenUnconnected=off
  wires:
  Add4/1 -> Switch/1
  Add1/1 -> Switch/3
  Add3/1 -> Switch1/3
  Add2/1 -> Switch1/1
  Switch/1 -> X_out_0/1
  Switch1/1 -> Y_out_0/1
  Add6/1 -> Switch2/3
  Add5/1 -> Switch2/1
  Switch2/1 -> Ang_out_0/1
  X_in_0/1 -> Shift Arithmetic/1, Add1/1, Add4/1
  Y_in_0/1 -> Shift Arithmetic1/1, Add3/1, Add2/1
  Ang_in_0/1 -> Add6/1, Add5/1, Compare To Constant/1
  Compare To Constant/1 -> Logical Operator1/1, Switch/2, Switch2/2
  Shift Arithmetic1/1 -> Add1/2, Add4/2
  Shift Arithmetic/1 -> Add3/2, Add2/2
  Logical Operator1/1 -> Switch1/2
  ANGLE/1 -> Add6/2, Add5/2

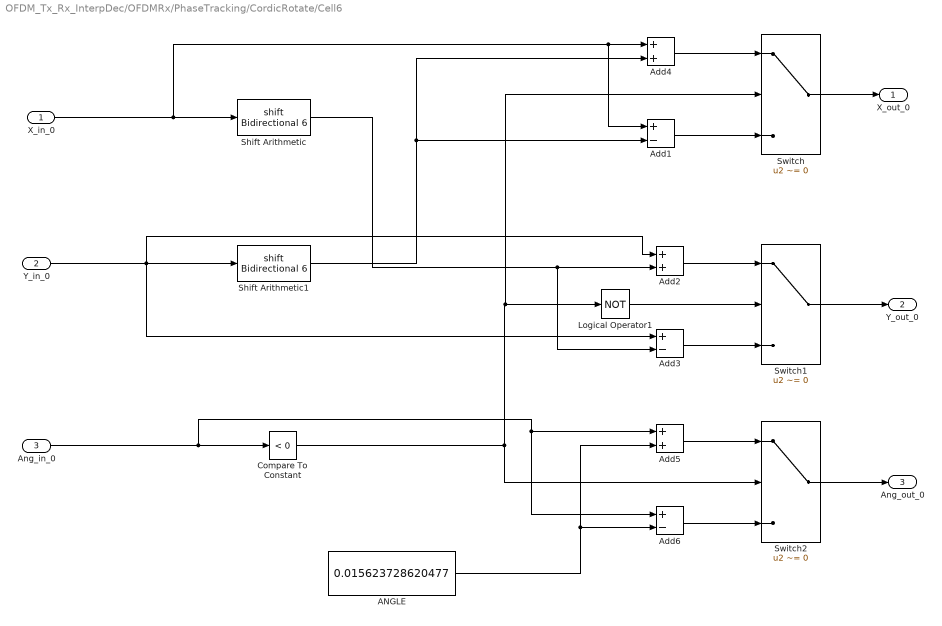
== system OFDM_Tx_Rx_InterpDec/OFDMRx/PhaseTracking/CordicRotate/Cell6 ==
  X_in_0 : Inport
  Y_in_0 : Inport  Port=2
  Ang_in_0 : Inport  Port=3
  ANGLE : Constant  Value=0.015623728620477  VectorParams1D=off  OutDataTypeStr=fixdt(1,23,20)  SampleTime=1/fs
  Add1 : Sum  Inputs=+-  OutDataTypeStr=fixdt(1,21,15)
  Add2 : Sum  OutDataTypeStr=fixdt(1,21,15)
  Add3 : Sum  Inputs=+-  OutDataTypeStr=fixdt(1,21,15)
  Add4 : Sum  OutDataTypeStr=fixdt(1,21,15)
  Add5 : Sum  OutDataTypeStr=fixdt(1,23,20)
  Add6 : Sum  Inputs=+-  OutDataTypeStr=fixdt(1,23,20)
  Compare To Constant : simulink/Logic and Bit Operations/Compare To Constant  relop=<  const=0  OutDataTypeStr=boolean
  Logical Operator1 : Logic  Operator=NOT  IconShape=distinctive  AllPortsSameDT=off  OutDataTypeStr=boolean
  Shift Arithmetic : ArithShift  BitShiftNumber=6
  Shift Arithmetic1 : ArithShift  BitShiftNumber=6
  Switch : Switch  Criteria=u2 ~= 0
  Switch1 : Switch  Criteria=u2 ~= 0
  Switch2 : Switch  Criteria=u2 ~= 0
  X_out_0 : Outport  VectorParamsAs1DForOutWhenUnconnected=off
  Y_out_0 : Outport  Port=2  VectorParamsAs1DForOutWhenUnconnected=off
  Ang_out_0 : Outport  Port=3  VectorParamsAs1DForOutWhenUnconnected=off
  wires:
  ANGLE/1 -> Add5/2, Add6/2
  Logical Operator1/1 -> Switch1/2
  Shift Arithmetic/1 -> Add2/2, Add3/2
  Shift Arithmetic1/1 -> Add4/2, Add1/2
  Compare To Constant/1 -> Switch2/2, Switch/2, Logical Operator1/1
  Ang_in_0/1 -> Compare To Constant/1, Add5/1, Add6/1
  Y_in_0/1 -> Add2/1, Add3/1, Shift Arithmetic1/1
  X_in_0/1 -> Add4/1, Add1/1, Shift Arithmetic/1
  Switch2/1 -> Ang_out_0/1
  Add5/1 -> Switch2/1
  Add6/1 -> Switch2/3
  Switch1/1 -> Y_out_0/1
  Switch/1 -> X_out_0/1
  Add2/1 -> Switch1/1
  Add3/1 -> Switch1/3
  Add1/1 -> Switch/3
  Add4/1 -> Switch/1

== system OFDM_Tx_Rx_InterpDec/OFDMRx/PhaseTracking/CordicRotate/Cell7 ==
  X_in_0 : Inport
  Y_in_0 : Inport  Port=2
  Ang_in_0 : Inport  Port=3
  ANGLE : Constant  Value=0.007812341060101  VectorParams1D=off  OutDataTypeStr=fixdt(1,23,20)  SampleTime=1/fs
  Add1 : Sum  Inputs=+-  OutDataTypeStr=fixdt(1,21,15)
  Add2 : Sum  OutDataTypeStr=fixdt(1,21,15)
  Add3 : Sum  Inputs=+-  OutDataTypeStr=fixdt(1,21,15)
  Add4 : Sum  OutDataTypeStr=fixdt(1,21,15)
  Add5 : Sum  OutDataTypeStr=fixdt(1,23,20)
  Add6 : Sum  Inputs=+-  OutDataTypeStr=fixdt(1,23,20)
  Compare To Constant : simulink/Logic and Bit Operations/Compare To Constant  relop=<  const=0  OutDataTypeStr=boolean
  Logical Operator1 : Logic  Operator=NOT  IconShape=distinctive  AllPortsSameDT=off  OutDataTypeStr=boolean
  Shift Arithmetic : ArithShift  BitShiftNumber=7
  Shift Arithmetic1 : ArithShift  BitShiftNumber=7
  Switch : Switch  Criteria=u2 ~= 0
  Switch1 : Switch  Criteria=u2 ~= 0
  Switch2 : Switch  Criteria=u2 ~= 0
  X_out_0 : Outport  VectorParamsAs1DForOutWhenUnconnected=off
  Y_out_0 : Outport  Port=2  VectorParamsAs1DForOutWhenUnconnected=off
  Ang_out_0 : Outport  Port=3  VectorParamsAs1DForOutWhenUnconnected=off
  wires:
  Add4/1 -> Switch/1
  Add1/1 -> Switch/3
  Add3/1 -> Switch1/3
  Add2/1 -> Switch1/1
  Switch/1 -> X_out_0/1
  Switch1/1 -> Y_out_0/1
  Add6/1 -> Switch2/3
  Add5/1 -> Switch2/1
  Switch2/1 -> Ang_out_0/1
  X_in_0/1 -> Shift Arithmetic/1, Add1/1, Add4/1
  Y_in_0/1 -> Shift Arithmetic1/1, Add3/1, Add2/1
  Ang_in_0/1 -> Add6/1, Add5/1, Compare To Constant/1
  Compare To Constant/1 -> Logical Operator1/1, Switch/2, Switch2/2
  Shift Arithmetic1/1 -> Add1/2, Add4/2
  Shift Arithmetic/1 -> Add3/2, Add2/2
  Logical Operator1/1 -> Switch1/2
  ANGLE/1 -> Add6/2, Add5/2

== system OFDM_Tx_Rx_InterpDec/OFDMRx/PhaseTracking/CordicRotate/Cell8 ==
  X_in_0 : Inport
  Y_in_0 : Inport  Port=2
  Ang_in_0 : Inport  Port=3
  ANGLE : Constant  Value=0.003906230131967  VectorParams1D=off  OutDataTypeStr=fixdt(1,23,20)  SampleTime=1/fs
  Add1 : Sum  Inputs=+-  OutDataTypeStr=fixdt(1,21,15)
  Add2 : Sum  OutDataTypeStr=fixdt(1,21,15)
  Add3 : Sum  Inputs=+-  OutDataTypeStr=fixdt(1,21,15)
  Add4 : Sum  OutDataTypeStr=fixdt(1,21,15)
  Add5 : Sum  OutDataTypeStr=fixdt(1,23,20)
  Add6 : Sum  Inputs=+-  OutDataTypeStr=fixdt(1,23,20)
  Compare To Constant : simulink/Logic and Bit Operations/Compare To Constant  relop=<  const=0  OutDataTypeStr=boolean
  Logical Operator1 : Logic  Operator=NOT  IconShape=distinctive  AllPortsSameDT=off  OutDataTypeStr=boolean
  Shift Arithmetic : ArithShift  BitShiftNumber=8
  Shift Arithmetic1 : ArithShift  BitShiftNumber=8
  Switch : Switch  Criteria=u2 ~= 0
  Switch1 : Switch  Criteria=u2 ~= 0
  Switch2 : Switch  Criteria=u2 ~= 0
  X_out_0 : Outport  VectorParamsAs1DForOutWhenUnconnected=off
  Y_out_0 : Outport  Port=2  VectorParamsAs1DForOutWhenUnconnected=off
  Ang_out_0 : Outport  Port=3  VectorParamsAs1DForOutWhenUnconnected=off
  wires:
  ANGLE/1 -> Add5/2, Add6/2
  Logical Operator1/1 -> Switch1/2
  Shift Arithmetic/1 -> Add2/2, Add3/2
  Shift Arithmetic1/1 -> Add4/2, Add1/2
  Compare To Constant/1 -> Switch2/2, Switch/2, Logical Operator1/1
  Ang_in_0/1 -> Compare To Constant/1, Add5/1, Add6/1
  Y_in_0/1 -> Add2/1, Add3/1, Shift Arithmetic1/1
  X_in_0/1 -> Add4/1, Add1/1, Shift Arithmetic/1
  Switch2/1 -> Ang_out_0/1
  Add5/1 -> Switch2/1
  Add6/1 -> Switch2/3
  Switch1/1 -> Y_out_0/1
  Switch/1 -> X_out_0/1
  Add2/1 -> Switch1/1
  Add3/1 -> Switch1/3
  Add1/1 -> Switch/3
  Add4/1 -> Switch/1

== system OFDM_Tx_Rx_InterpDec/OFDMRx/PhaseTracking/CordicRotate/Cell9 ==
  X_in_0 : Inport
  Y_in_0 : Inport  Port=2
  Ang_in_0 : Inport  Port=3
  ANGLE : Constant  Value=0.001953122516479  VectorParams1D=off  OutDataTypeStr=fixdt(1,23,20)  SampleTime=1/fs
  Add1 : Sum  Inputs=+-  OutDataTypeStr=fixdt(1,21,15)
  Add2 : Sum  OutDataTypeStr=fixdt(1,21,15)
  Add3 : Sum  Inputs=+-  OutDataTypeStr=fixdt(1,21,15)
  Add4 : Sum  OutDataTypeStr=fixdt(1,21,15)
  Add5 : Sum  OutDataTypeStr=fixdt(1,23,20)
  Add6 : Sum  Inputs=+-  OutDataTypeStr=fixdt(1,23,20)
  Compare To Constant : simulink/Logic and Bit Operations/Compare To Constant  relop=<  const=0  OutDataTypeStr=boolean
  Logical Operator1 : Logic  Operator=NOT  IconShape=distinctive  AllPortsSameDT=off  OutDataTypeStr=boolean
  Shift Arithmetic : ArithShift  BitShiftNumber=9
  Shift Arithmetic1 : ArithShift  BitShiftNumber=9
  Switch : Switch  Criteria=u2 ~= 0
  Switch1 : Switch  Criteria=u2 ~= 0
  Switch2 : Switch  Criteria=u2 ~= 0
  X_out_0 : Outport  VectorParamsAs1DForOutWhenUnconnected=off
  Y_out_0 : Outport  Port=2  VectorParamsAs1DForOutWhenUnconnected=off
  Ang_out_0 : Outport  Port=3  VectorParamsAs1DForOutWhenUnconnected=off
  wires:
  Add4/1 -> Switch/1
  Add1/1 -> Switch/3
  Add3/1 -> Switch1/3
  Add2/1 -> Switch1/1
  Switch/1 -> X_out_0/1
  Switch1/1 -> Y_out_0/1
  Add6/1 -> Switch2/3
  Add5/1 -> Switch2/1
  Switch2/1 -> Ang_out_0/1
  X_in_0/1 -> Shift Arithmetic/1, Add1/1, Add4/1
  Y_in_0/1 -> Shift Arithmetic1/1, Add3/1, Add2/1
  Ang_in_0/1 -> Add6/1, Add5/1, Compare To Constant/1
  Compare To Constant/1 -> Logical Operator1/1, Switch/2, Switch2/2
  Shift Arithmetic1/1 -> Add1/2, Add4/2
  Shift Arithmetic/1 -> Add3/2, Add2/2
  Logical Operator1/1 -> Switch1/2
  ANGLE/1 -> Add6/2, Add5/2

== system OFDM_Tx_Rx_InterpDec/OFDMRx/PhaseTracking/CordicRotate/GAIN_CORR ==
  XIN : Inport
  Constant : Constant  Value=0.607253321089875  OutDataTypeStr=fixdt(1,18,17)  SampleTime=1/fs
  Product : Product  OutDataTypeStr=fixdt(1,17,14)
  XOUT : Outport  VectorParamsAs1DForOutWhenUnconnected=off
  wires:
  Constant/1 -> Product/1
  XIN/1 -> Product/2
  Product/1 -> XOUT/1

== system OFDM_Tx_Rx_InterpDec/OFDMRx/PhaseTracking/CordicRotate/GAIN_CORR1 ==
  YIN : Inport
  Constant : Constant  Value=0.607253321089875  OutDataTypeStr=fixdt(1,18,17)  SampleTime=1/fs
  Product : Product  OutDataTypeStr=fixdt(1,17,14)
  YOUT : Outport  VectorParamsAs1DForOutWhenUnconnected=off
  wires:
  YIN/1 -> Product/2
  Constant/1 -> Product/1
  Product/1 -> YOUT/1

== system OFDM_Tx_Rx_InterpDec/OFDMRx/PhaseTracking/CordicRotate/QMAP ==
  X_in : Inport
  Y_in : Inport  Port=2
  Ctrl_in : Inport  Port=3
  QUAD_MAP1 : MATLAB Function  TreatAsAtomicUnit=on
  X_out : Outport  VectorParamsAs1DForOutWhenUnconnected=off
  Y_out : Outport  Port=2  VectorParamsAs1DForOutWhenUnconnected=off
  wires:
  QUAD_MAP1/2(yout) -> Y_out/1
  QUAD_MAP1/1(xout) -> X_out/1
  X_in/1 -> QUAD_MAP1/1(xin)
  Y_in/1 -> QUAD_MAP1/2(yin)
  Ctrl_in/1 -> QUAD_MAP1/3(ctrl)

== system OFDM_Tx_Rx_InterpDec/OFDMRx/PhaseTracking/CordicRotate/QUAD_MAP ==
  Xin : Inport
  Yin : Inport  Port=2
  ANG_IN : Inport  Port=3
  QUAD_DETERM1 : MATLAB Function  TreatAsAtomicUnit=on
  Xout : Outport  VectorParamsAs1DForOutWhenUnconnected=off
  Yout : Outport  Port=2  VectorParamsAs1DForOutWhenUnconnected=off
  ANG_OUT : Outport  Port=3  VectorParamsAs1DForOutWhenUnconnected=off
  QUAD_CTRL_OUT : Outport  Port=4  VectorParamsAs1DForOutWhenUnconnected=off
  wires:
  QUAD_DETERM1/2(QUAD) -> QUAD_CTRL_OUT/1
  Yin/1 -> Yout/1
  Xin/1 -> Xout/1
  QUAD_DETERM1/1(ang_out) -> ANG_OUT/1
  ANG_IN/1 -> QUAD_DETERM1/1(ang_in)

== system OFDM_Tx_Rx_InterpDec/OFDMRx/PhaseTracking/DataArrange/READ_CTRL ==
  In1 : Inport
  In2 : Inport  Port=2
  Constant : Constant  Value=0  OutDataTypeStr=fixdt(0,7,0)  SampleTime=1/fs
  Switch : Switch  Criteria=u2 ~= 0
  Out1 : Outport  VectorParamsAs1DForOutWhenUnconnected=off
  wires:
  Constant/1 -> Switch/3
  In2/1 -> Switch/2
  In1/1 -> Switch/1
  Switch/1 -> Out1/1

== system OFDM_Tx_Rx_InterpDec/OFDMRx/PhaseTracking/DataArrange/dataValidGen ==
  enb : Inport
  AND : Logic  IconShape=distinctive  AllPortsSameDT=off  OutDataTypeStr=boolean
  Compare To Constant : simulink/Logic and Bit Operations/Compare To Constant  relop=>  const=11  OutDataTypeStr=boolean
  HDL Counter2 : hdlsllib/Sources/HDL Counter  CountType=Count limited  CountInit=0  CountStep=1  CountMax=63  CountFromType=Initial value  CountFrom=0  CountResetPort=on  CountLoadPort=off  CountEnbPort=on  CountDirPort=off  CountDataType=Unsigned  CountWordLen=8  CountFracLen=0  CountSampTime=1
  NOT : Logic  Operator=NOT  IconShape=distinctive  AllPortsSameDT=off  OutDataTypeStr=boolean
  dataValidOut : Outport
  wires:
  NOT/1 -> HDL Counter2/1
  HDL Counter2/1 -> Compare To Constant/1
  enb/1 -> AND/2, NOT/1, HDL Counter2/2
  AND/1 -> dataValidOut/1
  Compare To Constant/1 -> AND/1

== system OFDM_Tx_Rx_InterpDec/OFDMRx/PhaseTracking/PhaseEst/CIC_MA ==
  In1 : Inport
  Add : Sum  Inputs=-+  AccumDataTypeStr=fixdt(1,23,15)
  Add1 : Sum  AccumDataTypeStr=fixdt(1,23,15)
  Delay1 : Delay  DelayLength=4
  Delay2 : Delay  DelayLength=1
  Out1 : Outport  VectorParamsAs1DForOutWhenUnconnected=off
  wires:
  Delay2/1 -> Out1/1, Add1/1
  In1/1 -> Delay1/1, Add/2
  Delay1/1 -> Add/1
  Add/1 -> Add1/2
  Add1/1 -> Delay2/1

== system OFDM_Tx_Rx_InterpDec/OFDMRx/PhaseTracking/PilotCtrlGen/CtrlSigGen ==
  valid : Inport
  sampleCount : Inport  Port=2
  Compare To Constant1 : simulink/Logic and Bit Operations/Compare To Constant  relop===  const=3  OutDataTypeStr=boolean
  Compare To Constant4 : simulink/Logic and Bit Operations/Compare To Constant  relop=>=  const=4  OutDataTypeStr=boolean
  Compare To Constant5 : simulink/Logic and Bit Operations/Compare To Constant  relop=<=  const=51  OutDataTypeStr=boolean
  Logical Operator2 : Logic  IconShape=distinctive  AllPortsSameDT=off  OutDataTypeStr=boolean
  Logical Operator4 : Logic  IconShape=distinctive  AllPortsSameDT=off  OutDataTypeStr=boolean
  Logical Operator5 : Logic  IconShape=distinctive  AllPortsSameDT=off  OutDataTypeStr=boolean
  dataValid : Outport
  pilotEnd : Outport  Port=2
  wires:
  Compare To Constant5/1 -> Logical Operator2/2
  Logical Operator5/1 -> pilotEnd/1
  Compare To Constant4/1 -> Logical Operator2/1
  Compare To Constant1/1 -> Logical Operator5/2
  Logical Operator2/1 -> Logical Operator4/2
  Logical Operator4/1 -> dataValid/1
  sampleCount/1 -> Compare To Constant1/1, Compare To Constant5/1, Compare To Constant4/1
  valid/1 -> Logical Operator4/1, Logical Operator5/1

== system OFDM_Tx_Rx_InterpDec/OFDMRx/PhaseTracking/PilotCtrlGen/SampleCounter ==
  Valid_In : Inport
  Delay : Delay  DelayLength=1
  Logical Operator : Logic  Operator=NOT  IconShape=distinctive  AllPortsSameDT=off  OutDataTypeStr=boolean
  SAMPLE_COUNTER : hdlsllib/Sources/HDL Counter  CountType=Count limited  CountInit=0  CountStep=1  CountMax=51  CountFromType=Initial value  CountFrom=0  CountResetPort=on  CountLoadPort=off  CountEnbPort=on  CountDirPort=off  CountDataType=Unsigned  CountWordLen=6  CountFracLen=0  CountSampTime=1
  Sample_Cnt : Outport  VectorParamsAs1DForOutWhenUnconnected=off
  wires:
  SAMPLE_COUNTER/1 -> Delay/1
  Valid_In/1 -> Logical Operator/1, SAMPLE_COUNTER/2
  Logical Operator/1 -> SAMPLE_COUNTER/1
  Delay/1 -> Sample_Cnt/1

== system OFDM_Tx_Rx_InterpDec/OFDMRx/PhaseTracking/PilotCtrlGen/SymbolCounter ==
  ValidIn : Inport
  Delay : Delay  DelayLength=1
  HDL Counter : hdlsllib/Sources/HDL Counter  CountType=Count limited  CountInit=0  CountStep=1  CountMax=126  CountFromType=Initial value  CountFrom=0  CountResetPort=off  CountLoadPort=off  CountEnbPort=on  CountDirPort=off  CountDataType=Unsigned  CountWordLen=7  CountFracLen=0  CountSampTime=1
  Relational Operator : RelationalOperator  Operator=<  OutDataTypeStr=boolean  RndMeth=Nearest
  Symbl_cnt : Outport  VectorParamsAs1DForOutWhenUnconnected=off
  wires:
  ValidIn/1 -> Relational Operator/1, Delay/1
  Delay/1 -> Relational Operator/2
  HDL Counter/1 -> Symbl_cnt/1
  Relational Operator/1 -> HDL Counter/1

== system OFDM_Tx_Rx_InterpDec/OFDMRx/PhaseTracking/PilotCtrlGen/pilotGen ==
  symbCount : Inport
  sampleCount : Inport  Port=2
  valid : Inport  Port=3
  Compare To Constant : simulink/Logic and Bit Operations/Compare To Constant  relop=>  const=0  OutDataTypeStr=boolean
  Compare To Constant2 : simulink/Logic and Bit Operations/Compare To Constant  relop=>=  const=0  OutDataTypeStr=boolean
  Compare To Constant3 : simulink/Logic and Bit Operations/Compare To Constant  relop=<  const=4  OutDataTypeStr=boolean
  Constant : Constant  Value=0  OutDataTypeStr=fixdt(1,2,0)  SampleTime=1/fs
  HDL Counter1 : hdlsllib/Sources/HDL Counter  CountType=Count limited  CountInit=0  CountStep=1  CountMax=3  CountFromType=Initial value  CountFrom=0  CountResetPort=off  CountLoadPort=off  CountEnbPort=on  CountDirPort=off  CountDataType=Unsigned  CountWordLen=2  CountFracLen=0  CountSampTime=1
  Logical Operator1 : Logic  IconShape=distinctive  AllPortsSameDT=off  OutDataTypeStr=boolean
  Logical Operator3 : Logic  IconShape=distinctive  AllPortsSameDT=off  OutDataTypeStr=boolean
  PilotValue_LUT1 : Lookup_n-D  NumberOfTableDimensions=1  LookupTableObject=''  BreakpointsForDimension1=[0:3]  BreakpointsForDimension1FirstPoint=10  BreakpointsForDimension2FirstPoint=10  BreakpointsForDimension1Spacing=12  BreakpointsForDimension2Spacing=12  IndexSearchMethod=Evenly spaced points  Table=[1 1 1 -1]  TableDataTypeStr=fixdt(1,2,0)  InterpMethod=Flat  DiagnosticForOutOfRangeInput=Error  InternalRulePriority=Speed  OutDataTypeStr=fixdt(1,2,0)  RndMeth=Simplest  InputSameDT=on
  Polarity_LUT1 : Lookup_n-D  NumberOfTableDimensions=1  LookupTableObject=''  BreakpointsForDimension1=[0:126]  BreakpointsForDimension1FirstPoint=10  BreakpointsForDimension2FirstPoint=10  BreakpointsForDimension1Spacing=12  BreakpointsForDimension2Spacing=12  IndexSearchMethod=Evenly spaced points  Table=pilot  TableDataTypeStr=fixdt(1,2,0)  InterpMethod=Flat  DiagnosticForOutOfRangeInput=Error  InternalRulePriority=Speed  OutDataTypeStr=fixdt(1,2,0)  RndMeth=Simplest  InputSameDT=on
  Switch : Switch  Criteria=u2 ~= 0
  Switch1 : Switch  Criteria=u2 ~= 0
  ToComplex1 : Subsystem
  Unary Minus : UnaryMinus
  pilOut : Outport
  wires:
  HDL Counter1/1 -> PilotValue_LUT1/1
  Polarity_LUT1/1 -> Compare To Constant/1
  PilotValue_LUT1/1 -> Switch1/1
  Switch/1 -> ToComplex1/1(In1)
  Unary Minus/1 -> Switch/3
  Compare To Constant/1 -> Switch/2
  ToComplex1/1(Out1) -> pilOut/1
  Switch1/1 -> Unary Minus/1, Switch/1
  Constant/1 -> Switch1/3
  symbCount/1 -> Polarity_LUT1/1
  sampleCount/1 -> Compare To Constant2/1, Compare To Constant3/1
  Logical Operator1/1 -> Logical Operator3/2
  Compare To Constant2/1 -> Logical Operator1/1
  Compare To Constant3/1 -> Logical Operator1/2
  valid/1 -> Logical Operator3/1
  Logical Operator3/1 -> Switch1/2, HDL Counter1/1

== system OFDM_Tx_Rx_InterpDec/OFDMRx/Synchronisation/CoarseFreqCorr/RsingEdge ==
  In1 : Inport
  Delay : Delay  DelayLength=1
  Relational Operator : RelationalOperator  Operator=>  OutDataTypeStr=boolean  RndMeth=Nearest
  Out1 : Outport  VectorParamsAs1DForOutWhenUnconnected=off
  wires:
  Relational Operator/1 -> Out1/1
  Delay/1 -> Relational Operator/2
  In1/1 -> Delay/1, Relational Operator/1

== system OFDM_Tx_Rx_InterpDec/OFDMRx/Synchronisation/CoarseTimingSynch/CoarseTimeStrobeGen ==
  dataIn : Inport
  packetDet : Inport  Port=2
  LocalSearchCounter : Subsystem
  MaxPeakDet : Subsystem
  coarseStrobeOut : Outport  VectorParamsAs1DForOutWhenUnconnected=off
  wires:
  LocalSearchCounter/1(coutEnb) -> MaxPeakDet/2(CntEnbIn)
  MaxPeakDet/1(CoarseStrbOut) -> coarseStrobeOut/1
  LocalSearchCounter/2(countOut) -> MaxPeakDet/3(CountIn)
  dataIn/1 -> MaxPeakDet/1(DataIn)
  packetDet/1 -> LocalSearchCounter/1(packDetIn)

== system OFDM_Tx_Rx_InterpDec/OFDMRx/Synchronisation/ControlSigGen/PreambleValidGen ==
  ValidIn : Inport
  Compare To Constant : simulink/Logic and Bit Operations/Compare To Constant  relop===  const=128  OutDataTypeStr=boolean
  HDL Counter : hdlsllib/Sources/HDL Counter  CountType=Count limited  CountInit=0  CountStep=1  CountMax=128  CountFromType=Initial value  CountFrom=0  CountResetPort=on  CountLoadPort=off  CountEnbPort=on  CountDirPort=off  CountDataType=Unsigned  CountWordLen=8  CountFracLen=0  CountSampTime=1
  NOT : Logic  Operator=NOT  IconShape=distinctive  AllPortsSameDT=off  OutDataTypeStr=boolean
  RisingEdge : Subsystem
  Unit Delay Enabled Resettable Synchronous : hdlsllib/Discrete/Unit Delay Enabled Resettable Synchronous  InitialCondition=0.0  SampleTime=-1
      settings: SourceProductBaseCode=SL
  y : Outport
  wires:
  Unit Delay Enabled Resettable Synchronous/1 -> y/1
  ValidIn/1 -> Unit Delay Enabled Resettable Synchronous/1, HDL Counter/2, NOT/1, RisingEdge/1(ValidIn)
  Compare To Constant/1 -> Unit Delay Enabled Resettable Synchronous/3
  NOT/1 -> HDL Counter/1
  RisingEdge/1(Out1) -> Unit Delay Enabled Resettable Synchronous/2
  HDL Counter/1 -> Compare To Constant/1
